simulink model "fsk_simulink"  (R2015a)
settings: Solver=ode45  StartTime=0.0  StopTime=10.0  RelTol=1e-3
settings Model: Creator=tatuapu  LastModifiedBy=tatuapu

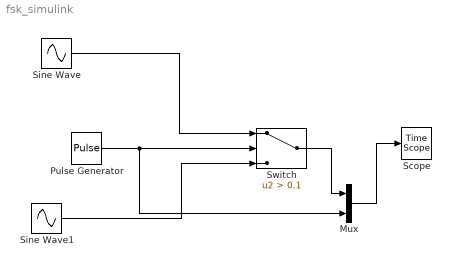
== system fsk_simulink ==
  Mux : Mux  Inputs=2
  Pulse Generator : DiscretePulseGenerator  PulseType=Time based  PulseWidth=50
  Scope : TimeScope
  Sine Wave : Sin  Frequency=500  SampleTime=0.001
  Sine Wave1 : Sin  Frequency=100  SampleTime=0.001
  Switch : Switch  Criteria=u2 > Threshold  Threshold=0.1
  wires:
  Pulse Generator/1 -> Mux/2, Switch/2
  Sine Wave/1 -> Switch/1
  Sine Wave1/1 -> Switch/3
  Switch/1 -> Mux/1
  Mux/1 -> Scope/1
